simulink model "MINI_BANSHEE"  (Simulink 8.1)
settings: Solver=ode1  StartTime=0.0  StopTime=inf  FixedStep=Ts  MaxStep=1e-3  RelTol=1e-3
model workspace (MAT data in the model file):
  op_snapshot1 : opcond.OperatingPoint (value not decoded)
PostLoadFcn:
  | BANSHEE_init;
InitFcn:
  | BANSHEE_init;
undefined symbols (not defined in the file): cable_spec, F1, F2, F3, fdesignblkfcn, gcbh, Left, SM_UtilityService, Ts, type, utility_service_lib, V
libraries: rtio_generic_modbus x21, relay_modbus_lib x20, cables_lib x19, breaker_lib x18, rtio_opalrt_common x15, rtlab x14, simulink x10, artemis x7, transformer_lib x7, simulink_extras x6, PQFV_lib x5, rtio_opalrt_op5142ex1 x4
(part 1 of 3)
settings Model: ARTEMISmethode_block_infos=$$__separator__$$MINI_BANSHEE/ARTEMIS Guide$$__separator__$$  Creator=RE25624  LastModifiedBy=re25624  BufferReuse=off
settings SolverCC: ZeroCrossAlgorithm=Adaptive
settings DataIOCC: ExternalInput=getinputstruct(op_snapshot1)  InitialState=getstatestruct(op_snapshot1)  LimitDataPoints=off  MaxDataPoints=90060  SignalLoggingSaveFormat=Dataset  SaveOutput=off  SignalLogging=off  DSMLogging=off  SaveTime=off  OutputSaveName=result
settings OptimizationCC: BlockReduction=off  OptimizeBlockIOStorage=off  BufferReuse=off  ExpressionFolding=off  LocalBlockOutputs=off
settings DebuggingCC: MaxConsecutiveZCsMsg=warning  IgnoredZcDiagnostic=none  SolverPrmCheckMsg=none  MultiTaskRateTransMsg=warning  FcnCallInpInsideContextMsg=EnableAllAsWarning  FrameProcessingCompatibilityMsg=error  ModelReferenceExtraNoncontSigs=warning  StrictBusMsg=None
settings ModelReferenceCC: UpdateModelReferenceTargets=IfOutOfDate
settings SFSimCC: SFSimEcho=off
settings GRTTargetCC: CodeReplacementLibrary=C89/C90 (ANSI)

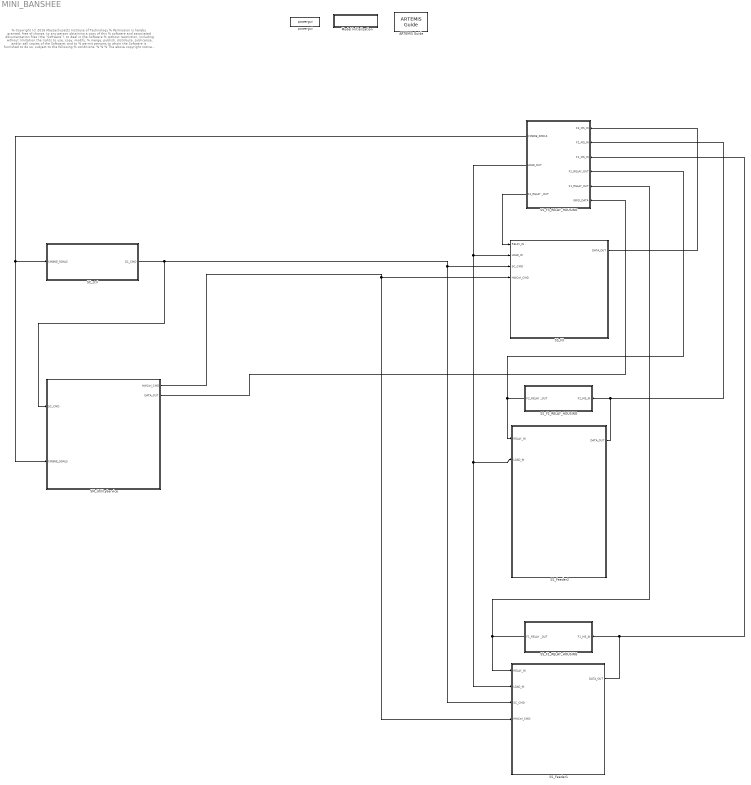
== system MINI_BANSHEE ==
  note: % Copyright (c) 2016 Massachusetts Institute of Technology
      | % Permission is hereby granted, free of charge, to any person obtaining a copy of this
      | % software and associated documentation files (the "Software"), to deal in the Software
      | % without restriction, including without limitation the rights to use, copy, modify,
      | % merge, publish, distribute, sublicense, and/or sell copies of the Software, and to
      | % permit persons to whom the Software is furnished to do so, subject to the following
      | % conditions:
      | %
      | %
      | % The above copyright notice and this permission notice shall be included in
      | % all copies or substantial portions of the Software.
      | %
      | % THE SOFTWARE IS PROVIDED "AS IS", WITHOUT WARRANTY OF ANY KIND, EXPRESS OR IMPLIED,
      | % INCLUDING BUT NOT LIMITED TO THE WARRANTIES OF MERCHANTABILITY, FITNESS FOR A
      | % PARTICULAR PURPOSE AND NONINFRINGEMENT. IN NO EVENT SHALL THE AUTHORS OR COPYRIGHT
      | % HOLDERS BE LIABLE FOR ANY CLAIM, DAMAGES OR OTHER LIABILITY, WHETHER IN AN ACTION
      | % OF CONTRACT, TORT OR OTHERWISE, ARISING FROM, OUT OF OR IN CONNECTION WITH THE
      | % SOFTWARE OR THE USE OR OTHER DEALINGS IN THE SOFTWARE.
      | %
      | %
      | %%
  ARTEMIS Guide : artemis/ARTEMIS/ARTEMIS Guide  Tag=FTSSmethode_opal_4hx0r99  Description=5.0_z1  lock=on  Ts=Ts  opt=art5  dyna=off  nb_perm=4  RT_fullcomp=off  ssn=on  ssn_itvc=off  ssn_ivic=off  ssn_ext=off  ssn_solver=Art5 with Backward Euler nodal interface  ssn_impulse=off  ssn_quasimpulse=off  ssn_impulse_loop=5  paraExtinctionThy=off  Thy_Impulse=on  dtc=Off  dtc_opt=normal  ao=on  simtype=off  ct_mac=off  lin_mov=off  lsp=[0.001 2]  spike_skip=Disabled  dtc_extra=1  dtc_sws=normal  dtc_pied=0.5  SPSRulesBlock=SPSRules  tre=on  ctmm=off  LF=off  dpl_type=ARTEMiS DPL  rlc_type=off  custom_type=off  para=on  ssn_ImpulseLoopBlockedStateUpdate=5  ssn_mov_iter_number=5  ssn_switch_iter_number=5
  Model Initialization : Subsystem  AncestorBlock=artemis/Tools /Misc/Model Initialization  mask(Model Functions){InitFcnX=BANSHEE_init;, prel=off, posl=on, inif=on, strf=off}
      mask prompts: InitFcnX "Initialisation"; prel "Preload Function"; posl "PostLoad Function"; inif "InitFcn"; strf "StartFcn"
      mask init:
      | currentBlock = gcb;
      | root = bdroot(currentBlock);
      | 
      | if ~strcmp(get_param(root,'BlockDiagramType'),'library')
      |     if prel==1
      |         set_param(root, 'PreLoadFcn', InitFcnX);
      |     else
      |         set_param(root, 'PreLoadFcn', '');
      |     end
      |     if inif==1
      |         set_param(root, 'InitFcn', InitFcnX);
      |     else
      |         set_param(root, 'InitFcn', '');
      |     end
      |     if strf==1
      |         set_param(root, 'StartFcn', InitFcnX);
      |     else
      |         set_param(root, 'StartFcn', '');
      |     end
      |     if posl==1
      |         set_param(root, 'PostLoadFcn', InitFcnX);
      |     else
      |         set_param(root, 'PostLoadFcn', '');
      |     end
      | end
      | 
      | pos = get_param(currentBlock, 'Position');
      | width = pos(3) - pos(1); height = pos(4) - pos(2);
      | txt = [ upper(root) '\n' '- InitFcn. . . . . '  get_param(root, 'InitFcn') ];
      settings: CopyFcn=set_param(gcb,'LinkStatus','inactive')
      mask Display: text(5, height*0.5, txt, 'horizontalAlignment', 'left', 'verticalAlignment', 'middle') ;
  SC_ctrl : Subsystem
  SM_UtilityService : Subsystem  AncestorBlock=utility_service_lib/SM_UtilityService
  SS_F1_RELAY_HOUSING : Subsystem
  SS_F2_RELAY_HOUSING : Subsystem
  SS_F3 : Subsystem
  SS_F3_RELAY_HOUSING : Subsystem
  SS_Feeder1 : Subsystem
  SS_Feeder2 : Subsystem
  powergui : powerlib/powergui  Priority=2  SimulationMode=Discrete  SolverType=Tustin  SampleTime=Ts  frequency=60  SPID=off  DisableSnubberDevices=off  DisableRonSwitches=off  DisableVfSwitches=off  SwTol=0  Interpol=off  DisplayEquations=off  frequencyindice=0  Pbase=100e6  ErrMax=1e-4  Iterations=50  UnitsV=kV  UnitsW=MW  FunctionMessages=off  echomessages=off  HookPort=off  EnableUseOfTLC=off  x0status=blocks  RestoreLinks=warning  ResistiveCurrentMeasurement=off  Frange=logspace(0,3,50)  Ylog=off  Xlog=off  ShowGrid=off  save=off  variable=ZData  structure=0  ZoomFFT=on  StartTime=0.0  cycles=2  DisplayStyle=off  fundamental=60  FreqAxis=off  MaxFrequency=1000  frequencyindicesteady=1  RmsSteady=1  display=off  Ts=0  methode=off
  wires:
  SS_F3/1(DATA_OUT) -> SS_F3_RELAY_HOUSING/1(F3_MS_IN)
  SS_F3_RELAY_HOUSING/3(F3_RELAY _OUT) -> SS_F3/1(RELAY_IN)
  SS_F1_RELAY_HOUSING/1(F1_RELAY _OUT) -> SS_Feeder1/1(RELAY_IN), SS_F3_RELAY_HOUSING/5(F1_RELAY_OUT)
  SS_F2_RELAY_HOUSING/1(F2_RELAY _OUT) -> SS_F3_RELAY_HOUSING/4(F2_RELAY_OUT), SS_Feeder2/1(RELAY_IN)
  SS_Feeder1/1(DATA_OUT) -> SS_F3_RELAY_HOUSING/3(F1_MS_IN), SS_F1_RELAY_HOUSING/1(F1_MS_IN)
  SS_Feeder2/1(DATA_OUT) -> SS_F3_RELAY_HOUSING/2(F2_MS_IN), SS_F2_RELAY_HOUSING/1(F2_MS_IN)
  SM_UtilityService/2(DATA_OUT) -> SS_F3_RELAY_HOUSING/6(GRID_DATA)
  SC_ctrl/1(SC_CMD) -> SM_UtilityService/1(SC_CMD), SS_Feeder1/3(SC_CMD), SS_F3/3(SC_CMD)
  SS_F3_RELAY_HOUSING/2(LOAD_OUT) -> SS_F3/2(LOAD_IN), SS_Feeder1/2(LOAD_IN), SS_Feeder2/2(LOAD_IN)
  SM_UtilityService/1(HWCtrl_CMD) -> SS_Feeder1/4(HWCtrl_CMD), SS_F3/4(HWCtrl_CMD)
  SS_F3_RELAY_HOUSING/1(CMBNE_SGNLS) -> SM_UtilityService/2(CMBNE_SGNLS), SC_ctrl/1(CMBNE_SGNLS)

== system MINI_BANSHEE/Model Initialization ==

== system MINI_BANSHEE/SC_ctrl ==
  note: % Copyright (c) 2016 Massachusetts Institute of Technology
      | % Permission is hereby granted, free of charge, to any person obtaining a copy of this
      | % software and associated documentation files (the "Software"), to deal in the Software
      | % without restriction, including without limitation the rights to use, copy, modify,
      | % merge, publish, distribute, sublicense, and/or sell copies of the Software, and to
      | % permit persons to whom the Software is furnished to do so, subject to the following
      | % conditions:
      | %
      | %
      | % The above copyright notice and this permission notice shall be included in
      | % all copies or substantial portions of the Software.
      | %
      | % THE SOFTWARE IS PROVIDED "AS IS", WITHOUT WARRANTY OF ANY KIND, EXPRESS OR IMPLIED,
      | % INCLUDING BUT NOT LIMITED TO THE WARRANTIES OF MERCHANTABILITY, FITNESS FOR A
      | % PARTICULAR PURPOSE AND NONINFRINGEMENT. IN NO EVENT SHALL THE AUTHORS OR COPYRIGHT
      | % HOLDERS BE LIABLE FOR ANY CLAIM, DAMAGES OR OTHER LIABILITY, WHETHER IN AN ACTION
      | % OF CONTRACT, TORT OR OTHERWISE, ARISING FROM, OUT OF OR IN CONNECTION WITH THE
      | % SOFTWARE OR THE USE OR OTHER DEALINGS IN THE SOFTWARE.
      | %
      | %
      | %%
  note: The 'Overruns' value should remain at 0.
      | The 'Ttotal' value should be equal to the
      | model Fixed-Step size.
  CMBNE_SGNLS : Inport
  Bus Creator : BusCreator  Inputs=2
  Bus Creator1 : BusCreator  Inputs=3
  Bus Selector : BusSelector  OutputSignals=F1_RELAY_OUT,F2_RELAY_OUT,F3_RELAY_OUT
  F1 1: connect motor 0: disconnect motor1 : Constant  Value=0
  F3 1: connect motor 0: disconnect motor : Constant  Value=0
  OpComm : rtlab/OpComm  nbport=1  groupe_acq=1  subsys_rate=0  st=0  Synchronization=on  Interpolation=on  Threshold=1.0  Missed_Data=off  Sim_Time=off  Samples=off  dynSigOut=off  from_console=0  warning_done=off  writeOpCommFile=off  Offset=off
  Overall : Subsystem
  Status : Subsystem
  Woodward : Subsystem
  opElectricFaultSelector : artemis/Tools /POW faults/opElectricFaultSelector  phase_a=on  phase_b=on  phase_c=on  gnd_fault=on  Tacq=1  Tst=[0.1 0 10]  enable_POW=off  angle_POW=[15 0 10]  Tdr="[0.5 0  10]"  fault_location_menu=No fault  T_init=2
  SC_CMD : Outport
  wires:
  CMBNE_SGNLS/1 -> OpComm/1
  Bus Selector/1 -> Overall/1(F1), Status/1(F1)  "<F1_RELAY_OUT>"
  Bus Selector/2 -> Overall/2(F2), Status/2(F2)  "<F2_RELAY_OUT>"
  Bus Selector/3 -> Status/3(F3), Overall/3(F3)  "<F3_RELAY_OUT>"
  opElectricFaultSelector/1 -> [fault_cmd]
  Bus Creator1/1 -> SC_CMD/1
  [IO_ctrl] -> Bus Creator1/3  "IO ctrl"
  Woodward/1(IOctrl) -> [IO_ctrl]
  [fault_cmd] -> Bus Creator1/1  "fault_cmd"
  OpComm/1 -> Bus Selector/1
  Bus Creator/1 -> Bus Creator1/2  "motor_ONOFF"
  F3 1: connect motor 0: disconnect motor/1 -> Bus Creator/1  "F3_motor_ONOFF"
  F1 1: connect motor 0: disconnect motor1/1 -> Bus Creator/2  "F1_motor_ONOFF"

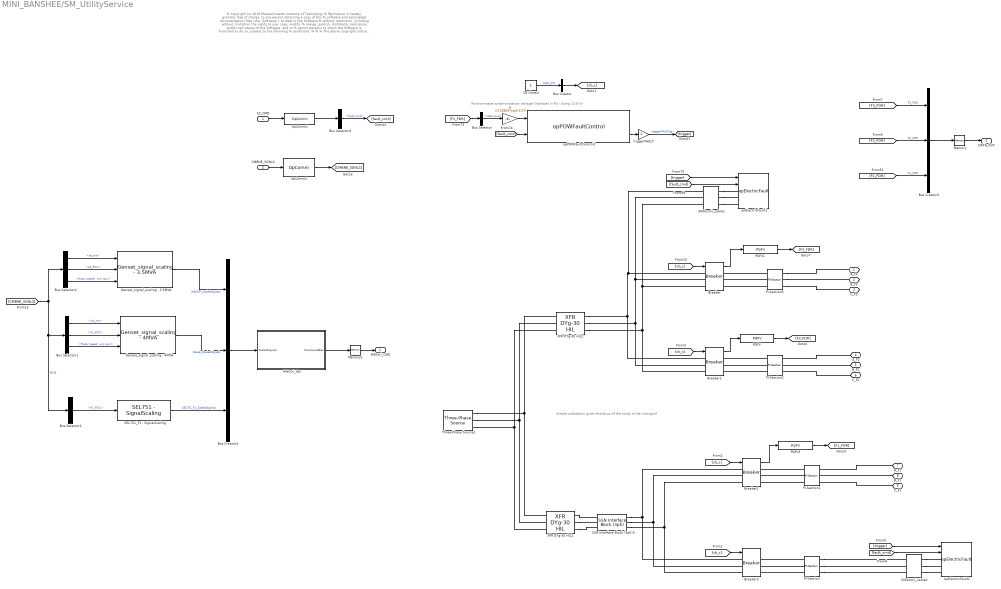
== system MINI_BANSHEE/SM_UtilityService ==
  note: Simple substation given the focus of the study is the microgrid
  note: % Copyright (c) 2016 Massachusetts Institute of Technology
      | % Permission is hereby granted, free of charge, to any person obtaining a copy of this
      | % software and associated documentation files (the "Software"), to deal in the Software
      | % without restriction, including without limitation the rights to use, copy, modify,
      | % merge, publish, distribute, sublicense, and/or sell copies of the Software, and to
      | % permit persons to whom the Software is furnished to do so, subject to the following
      | % conditions:
      | %
      | %
      | % The above copyright notice and this permission notice shall be included in
      | % all copies or substantial portions of the Software.
      | %
      | % THE SOFTWARE IS PROVIDED "AS IS", WITHOUT WARRANTY OF ANY KIND, EXPRESS OR IMPLIED,
      | % INCLUDING BUT NOT LIMITED TO THE WARRANTIES OF MERCHANTABILITY, FITNESS FOR A
      | % PARTICULAR PURPOSE AND NONINFRINGEMENT. IN NO EVENT SHALL THE AUTHORS OR COPYRIGHT
      | % HOLDERS BE LIABLE FOR ANY CLAIM, DAMAGES OR OTHER LIABILITY, WHETHER IN AN ACTION
      | % OF CONTRACT, TORT OR OTHERWISE, ARISING FROM, OUT OF OR IN CONNECTION WITH THE
      | % SOFTWARE OR THE USE OR OTHER DEALINGS IN THE SOFTWARE.
      | %
      | %
      | %%
  note: Point-on-wave synchronisation voltage (3-phase) in PU - Using 13.8 kV
  SC_CMD : Inport
  CMBNE_SGNLS : Inport  Port=2
  500kcmil_cable1 : cables_lib/500kcmil_cable  length=1  par_sets=1
  500kcmil_cable2 : cables_lib/500kcmil_cable  length=1  par_sets=1
  Breaker{,1..3} (4 alike) : breaker_lib/Breaker  Ts=Ts  mech_delay=cb_mech_delay
  Bus Creator : BusCreator  Inputs=1
  Bus Creator2 : BusCreator  Inputs=3
  Bus Creator4 : BusCreator  Inputs=3
  Bus Selector : BusSelector  OutputSignals=cb_ms.Vabc_bus
  Bus Selector1 : BusSelector  OutputSignals="F1_MS_IN.DIESEL_DATA.DIESEL_GCB.cb_ms,F1_MS_IN.CB_DATA.F1_PCC,F1_MS_IN.DIESEL_DATA.Gen2_meas.w.w.Rotor speed  wm (pu)"
  Bus Selector2 : BusSelector  OutputSignals=F1_MS_IN.CB_DATA.F1_PCC
  Bus Selector3 : BusSelector  OutputSignals=fault_cmd
  Bus Selector4 : BusSelector  OutputSignals="F3_MS_IN.NG_CHP_DATA.NG_CHP_GCB.cb_ms,F3_MS_IN.CB_DATA.F3_PCC,F3_MS_IN.NG_CHP_DATA.Gen1_meas.w.w.Rotor speed  wm (pu)"
  CB closed : Constant
  Genset_signal_scaling - 3.5MVA : EasyGen3500_GensetSignalScaling_lib/Genset_signal_scaling - 3.5MVA  Vpk_mcb=11268  watt_mcb=3150000  Vpk_gcb=11268  watt_gcb=3150000  rated_rpm=1800  wm_noise_bias=0.02
  Genset_signal_scaling - 4MVA : EasyGen3500_GensetSignalScaling_lib/Genset_signal_scaling - 4MVA  Vpk_mcb=11268  watt_mcb=3600000  Vpk_gcb=11268  watt_gcb=3600000  rated_rpm=1800  wm_noise_bias=0.02
  HWCtrl_IOs : Subsystem
  Memory : Memory
  Memory1 : Memory
  OpComm1 : rtlab/OpComm  nbport=1  groupe_acq=1  subsys_rate=0  st=0  Synchronization=on  Interpolation=on  Threshold=1.0  Missed_Data=off  Sim_Time=off  Samples=off  dynSigOut=off  from_console=1  warning_done=off  writeOpCommFile=off  Offset=off
  OpComm2 : rtlab/OpComm  nbport=1  groupe_acq=1  subsys_rate=0  st=0  Synchronization=on  Interpolation=on  Threshold=1.0  Missed_Data=off  Sim_Time=off  Samples=off  dynSigOut=off  from_console=0  warning_done=off  writeOpCommFile=off  Offset=off
  PI-Section : cables_lib/PI-Section  cable_spec=[cable_spec(13, :)]  line_length=3000  parallel_sets=1
  PI-Section1 : cables_lib/PI-Section  cable_spec=[cable_spec(13, :)]  line_length=500  parallel_sets=1
  PI-Section2 : cables_lib/PI-Section  cable_spec=[cable_spec(13, :)]  line_length=500  parallel_sets=1
  PI-Section3 : cables_lib/PI-Section  cable_spec=[cable_spec(13, :)]  line_length=500  parallel_sets=1
  PQFV : PQFV_lib/PQFV  VRMSLL=13800
  PQFV1 : PQFV_lib/PQFV  VRMSLL=13800
  PQFV3 : PQFV_lib/PQFV  VRMSLL=13800
  SEL751_F1 - SignalScaling : SEL751_SignalScaling_lib/SEL751 - SignalScaling  ct_ratio=1/1250  pt_ratio=1/1800
  SSN Interface Block (3ph)3 : ssn_lib/SSN Interface Block (3ph)  nb_phase=3  nb_port=2  p1_type=V-type(Left)  p2_type=V-type (Right)  p3_type=V-type(Left)  p4_type=V-type(Left)  p5_type=V-type(Left)  p6_type=V-type(Left)  p7_type=V-type(Left)  p8_type=V-type(Left)  p9_type=V-type(Left)  p10_type=V-type(Left)  p11_type=V-type(Left)  p12_type=V-type(Left)  p13_type=V-type(Left)  p14_type=V-type(Left)  p15_type=V-type(Left)  p16_type=V-type(Left)  I_port_shunt_resistance=1e9
  Three-Phase Source1 : powerlib/Electrical Sources/Three-Phase Source  Voltage=115000  PhaseAngle=0  Frequency=60  InternalConnection=Yg  SpecifyImpedance=on  Resistance=0.8929  Inductance=16.58e-3  ShortCircuitLevel=100e6  BaseVoltage=115000  XRratio=30  BusType=swing  Pref=0  Qref=0  Qmin=-inf  Qmax=inf
  XFR DYg-30 HIL1 : transformer_lib/XFR DYg-30 HIL  Rating=50000  Vp=115000  Vs=13800  Z=15  XR=30
  XFR DYg-30 HIL2 : transformer_lib/XFR DYg-30 HIL  Rating=50000  Vp=115000  Vs=13800  Z=15  XR=30
  a : Gain  Gain=1/(13800*sqrt(2/3))
  opElectricFault1 : artemis/Tools /POW faults/opElectricFault  FaultLocation=location 7  FaultResistance=0.0001  GroundResistance=0.0001  InitialStates=[0 0 0]  SnubberResistance=1e6  SnubberCapacitance=inf
  opElectricFault2 : artemis/Tools /POW faults/opElectricFault  FaultLocation=location 8  FaultResistance=0.0001  GroundResistance=0.0001  InitialStates=[0 0 0]  SnubberResistance=1e6  SnubberCapacitance=inf
  opPOWFaultControl1 : artemis/Tools /POW faults/opPOWFaultControl  Ts=Ts  usePLL=off  Fgrid=60  PLL_k=[180 3200 1]  vol_sel=1: rising zero-corssing  SyncPhase_menu=A  T_acq=0.8
  triggerFAULT : Gain
  A_F3 : PMIOPort  Port=1  Side=Right
  B_F3 : PMIOPort  Port=2  Side=Right
  C_F3 : PMIOPort  Port=3  Side=Right
  A_F2 : PMIOPort  Port=4  Side=Right
  B_F2 : PMIOPort  Port=5  Side=Right
  C_F2 : PMIOPort  Port=6  Side=Right
  A_F1 : PMIOPort  Port=7  Side=Right
  B_F1 : PMIOPort  Port=8  Side=Right
  C_F1 : PMIOPort  Port=9  Side=Right
  HWCtrl_CMD : Outport
  DATA_OUT : Outport  Port=2
  wires:
  [cb_c] -> Breaker2/1
  [cb_c] -> Breaker/1
  [cb_c] -> Breaker1/1
  [cb_c] -> Breaker3/1
  Bus Creator/1 -> [cb_c]
  CB closed/1 -> Bus Creator/1  "Logic_trip"
  [fault_cmd] -> opElectricFault1/2
  [trigger] -> opElectricFault1/1
  [fault_cmd] -> opPOWFaultControl1/2
  opPOWFaultControl1/2 -> triggerFAULT/1
  triggerFAULT/1 -> [trigger]  "triggerFAULTsig"
  [F1_FDR] -> Bus Selector/1
  Bus Selector/1 -> a/1  "<Vabc_bus>"
  a/1 -> opPOWFaultControl1/1
  [fault_cmd] -> opElectricFault2/2
  [trigger] -> opElectricFault2/1
  SC_CMD/1 -> OpComm1/1
  OpComm1/1 -> Bus Selector3/1
  Bus Selector3/1 -> [fault_cmd]  "<fault_cmd>"
  Memory1/1 -> HWCtrl_CMD/1
  Genset_signal_scaling - 3.5MVA/1 -> Bus Creator4/1  "NGCHP_ScaledSignals"
  Genset_signal_scaling - 4MVA/1 -> Bus Creator4/2  "Diesel_ScaledSignals"
  [CMBNE_SGNLS] -> Bus Selector4/1, Bus Selector2/1, Bus Selector1/1  "MCB"
  Bus Selector4/3 -> Genset_signal_scaling - 3.5MVA/3  "<Rotor speed  wm (pu)>"
  Bus Selector4/2 -> Genset_signal_scaling - 3.5MVA/2  "<F3_PCC>"
  Bus Selector4/1 -> Genset_signal_scaling - 3.5MVA/1  "<cb_ms>"
  Bus Creator4/1 -> HWCtrl_IOs/1(ScaledSignals)
  HWCtrl_IOs/1(WoodwardBias) -> Memory1/1
  Bus Selector1/3 -> Genset_signal_scaling - 4MVA/3  "<Rotor speed  wm (pu)>"
  Bus Selector1/2 -> Genset_signal_scaling - 4MVA/2  "<F1_PCC>"
  Bus Selector1/1 -> Genset_signal_scaling - 4MVA/1  "<cb_ms>"
  CMBNE_SGNLS/1 -> OpComm2/1
  OpComm2/1 -> [CMBNE_SGNLS]
  Breaker/1 -> PQFV1/1
  Breaker1/1 -> PQFV/1
  Breaker2/1 -> PQFV3/1
  PQFV3/1 -> [F1_FDR]
  PQFV1/1 -> [F3_FDR]
  PQFV/1 -> [F2_FDR]
  Memory/1 -> DATA_OUT/1
  Bus Creator2/1 -> Memory/1
  [F3_FDR] -> Bus Creator2/1  "F3_FDR"
  [F2_FDR] -> Bus Creator2/2  "F2_FDR"
  [F1_FDR] -> Bus Creator2/3  "F1_FDR"
  SEL751_F1 - SignalScaling/1 -> Bus Creator4/3  "SEL751_F1_ScaledSignals"
  Bus Selector2/1 -> SEL751_F1 - SignalScaling/1  "<F1_PCC>"
  connections:
  PI-Section2/LConn1 -- Breaker1/RConn1
  PI-Section2/LConn3 -- Breaker1/RConn3
  PI-Section1/LConn1 -- Breaker2/RConn1
  PI-Section1/LConn2 -- Breaker2/RConn2
  PI-Section3/LConn1 -- Breaker/RConn1
  PI-Section1/LConn3 -- Breaker2/RConn3
  Breaker3/LConn2 -- SSN Interface Block (3ph)3/RConn2 -- Breaker2/LConn2
  PI-Section3/LConn2 -- Breaker/RConn2
  Breaker3/LConn3 -- SSN Interface Block (3ph)3/RConn3 -- Breaker2/LConn3
  PI-Section/LConn3 -- Breaker3/RConn3
  PI-Section2/LConn2 -- Breaker1/RConn2
  PI-Section/LConn1 -- Breaker3/RConn1
  Breaker3/LConn1 -- SSN Interface Block (3ph)3/RConn1 -- Breaker2/LConn1
  PI-Section3/LConn3 -- Breaker/RConn3
  Breaker1/LConn2 -- 500kcmil_cable1/LConn2 -- Breaker/LConn2 -- XFR DYg-30 HIL2/RConn2
  XFR DYg-30 HIL2/RConn1 -- Breaker1/LConn1 -- 500kcmil_cable1/LConn1 -- Breaker/LConn1
  Breaker1/LConn3 -- 500kcmil_cable1/LConn3 -- Breaker/LConn3 -- XFR DYg-30 HIL2/RConn3
  PI-Section/LConn2 -- Breaker3/RConn2
  A_F2/RConn1 -- PI-Section2/RConn1
  B_F1/RConn1 -- PI-Section1/RConn2
  PI-Section3/RConn3 -- C_F3/RConn1
  Three-Phase Source1/RConn3 -- XFR DYg-30 HIL2/LConn3 -- XFR DYg-30 HIL1/LConn3
  Three-Phase Source1/RConn2 -- XFR DYg-30 HIL2/LConn2 -- XFR DYg-30 HIL1/LConn2
  Three-Phase Source1/RConn1 -- XFR DYg-30 HIL2/LConn1 -- XFR DYg-30 HIL1/LConn1
  C_F2/RConn1 -- PI-Section2/RConn3
  PI-Section3/RConn1 -- A_F3/RConn1
  B_F2/RConn1 -- PI-Section2/RConn2
  A_F1/RConn1 -- PI-Section1/RConn1
  C_F1/RConn1 -- PI-Section1/RConn3
  PI-Section3/RConn2 -- B_F3/RConn1
  500kcmil_cable1/RConn3 -- opElectricFault1/LConn3
  500kcmil_cable1/RConn2 -- opElectricFault1/LConn2
  500kcmil_cable1/RConn1 -- opElectricFault1/LConn1
  500kcmil_cable2/RConn3 -- opElectricFault2/LConn3
  500kcmil_cable2/RConn2 -- opElectricFault2/LConn2
  500kcmil_cable2/RConn1 -- opElectricFault2/LConn1
  PI-Section/RConn3 -- 500kcmil_cable2/LConn3
  PI-Section/RConn2 -- 500kcmil_cable2/LConn2
  PI-Section/RConn1 -- 500kcmil_cable2/LConn1
  XFR DYg-30 HIL1/RConn3 -- SSN Interface Block (3ph)3/LConn3
  XFR DYg-30 HIL1/RConn2 -- SSN Interface Block (3ph)3/LConn2
  XFR DYg-30 HIL1/RConn1 -- SSN Interface Block (3ph)3/LConn1

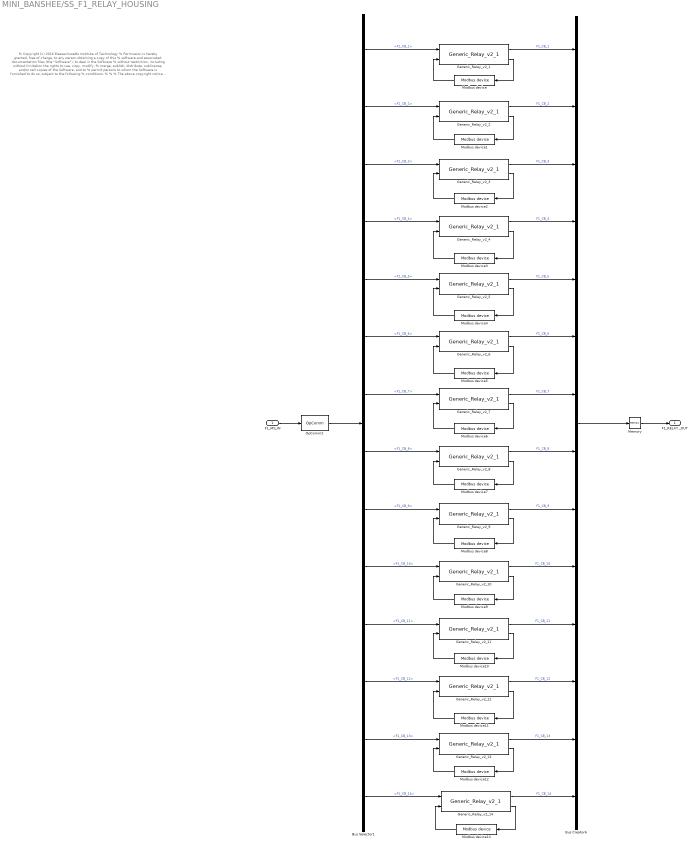
== system MINI_BANSHEE/SS_F1_RELAY_HOUSING ==
  note: % Copyright (c) 2016 Massachusetts Institute of Technology
      | % Permission is hereby granted, free of charge, to any person obtaining a copy of this
      | % software and associated documentation files (the "Software"), to deal in the Software
      | % without restriction, including without limitation the rights to use, copy, modify,
      | % merge, publish, distribute, sublicense, and/or sell copies of the Software, and to
      | % permit persons to whom the Software is furnished to do so, subject to the following
      | % conditions:
      | %
      | %
      | % The above copyright notice and this permission notice shall be included in
      | % all copies or substantial portions of the Software.
      | %
      | % THE SOFTWARE IS PROVIDED "AS IS", WITHOUT WARRANTY OF ANY KIND, EXPRESS OR IMPLIED,
      | % INCLUDING BUT NOT LIMITED TO THE WARRANTIES OF MERCHANTABILITY, FITNESS FOR A
      | % PARTICULAR PURPOSE AND NONINFRINGEMENT. IN NO EVENT SHALL THE AUTHORS OR COPYRIGHT
      | % HOLDERS BE LIABLE FOR ANY CLAIM, DAMAGES OR OTHER LIABILITY, WHETHER IN AN ACTION
      | % OF CONTRACT, TORT OR OTHERWISE, ARISING FROM, OUT OF OR IN CONNECTION WITH THE
      | % SOFTWARE OR THE USE OR OTHER DEALINGS IN THE SOFTWARE.
      | %
      | %
      | %%
  F1_MS_IN : Inport
  Bus Creator6 : BusCreator  Inputs=14
  Bus Selector1 : BusSelector  OutputSignals=CB_DATA.F1_CB_1,CB_DATA.F1_CB_2,CB_DATA.F1_CB_3,CB_DATA.F1_CB_4,CB_DATA.F1_CB_5,CB_DATA.F1_CB_6,CB_DATA.F1_CB_7,CB_DATA.F1_CB_8,CB_DATA.F1_CB_9,CB_DATA.F1_CB_10,CB_DATA.F1_CB_11,CB_DATA.F1_CB_12,CB_DATA.F1_CB_13,CB_DATA.F1_CB_14
  Generic_Relay_v2_1 : relay_modbus_lib/Generic_Relay_v2_1  Ts=Ts  relay_settings=[F1(1,:)]
  Generic_Relay_v2_10 : relay_modbus_lib/Generic_Relay_v2_1  Ts=Ts  relay_settings=[F1(10,:)]
  Generic_Relay_v2_11 : relay_modbus_lib/Generic_Relay_v2_1  Ts=Ts  relay_settings=[F1(11,:)]
  Generic_Relay_v2_12 : relay_modbus_lib/Generic_Relay_v2_1  Ts=Ts  relay_settings=[F1(12,:)]
  Generic_Relay_v2_13 : relay_modbus_lib/Generic_Relay_v2_1  Ts=Ts  relay_settings=[F1(13,:)]
  Generic_Relay_v2_14 : relay_modbus_lib/Generic_Relay_v2_1  Ts=Ts  relay_settings=[F1(14,:)]
  Generic_Relay_v2_2 : relay_modbus_lib/Generic_Relay_v2_1  Ts=Ts  relay_settings=[F1(2,:)]
  Generic_Relay_v2_3 : relay_modbus_lib/Generic_Relay_v2_1  Ts=Ts  relay_settings=[F1(3,:)]
  Generic_Relay_v2_4 : relay_modbus_lib/Generic_Relay_v2_1  Ts=Ts  relay_settings=[F1(4,:)]
  Generic_Relay_v2_5 : relay_modbus_lib/Generic_Relay_v2_1  Ts=Ts  relay_settings=[F1(5,:)]
  Generic_Relay_v2_6 : relay_modbus_lib/Generic_Relay_v2_1  Ts=Ts  relay_settings=[F1(6,:)]
  Generic_Relay_v2_7 : relay_modbus_lib/Generic_Relay_v2_1  Ts=Ts  relay_settings=[F1(7,:)]
  Generic_Relay_v2_8 : relay_modbus_lib/Generic_Relay_v2_1  Ts=Ts  relay_settings=[F1(8,:)]
  Generic_Relay_v2_9 : relay_modbus_lib/Generic_Relay_v2_1  Ts=Ts  relay_settings=[F1(9,:)]
  Memory : Memory
  Modbus device : rtio_generic_modbus/Modbus device  conf_name=F1_relay_cfg1.opal  conf_name_mask=F1_relay_cfg1.xls  sample_time=Ts
  Modbus device1 : rtio_generic_modbus/Modbus device  conf_name=F1_relay_cfg2.opal  conf_name_mask=F1_relay_cfg2.xls  sample_time=Ts
  Modbus device10 : rtio_generic_modbus/Modbus device  conf_name=F1_relay_cfg11.opal  conf_name_mask=F1_relay_cfg11.xls  sample_time=Ts
  Modbus device11 : rtio_generic_modbus/Modbus device  conf_name=F1_relay_cfg12.opal  conf_name_mask=F1_relay_cfg12.xls  sample_time=Ts
  Modbus device12 : rtio_generic_modbus/Modbus device  conf_name=F1_relay_cfg13.opal  conf_name_mask=F1_relay_cfg13.xls  sample_time=Ts
  Modbus device13 : rtio_generic_modbus/Modbus device  conf_name=F1_relay_cfg14.opal  conf_name_mask=F1_relay_cfg14.xls  sample_time=Ts
  Modbus device2 : rtio_generic_modbus/Modbus device  conf_name=F1_relay_cfg3.opal  conf_name_mask=F1_relay_cfg3.xls  sample_time=Ts
  Modbus device3 : rtio_generic_modbus/Modbus device  conf_name=F1_relay_cfg4.opal  conf_name_mask=F1_relay_cfg4.xls  sample_time=Ts
  Modbus device4 : rtio_generic_modbus/Modbus device  conf_name=F1_relay_cfg5.opal  conf_name_mask=F1_relay_cfg5.xls  sample_time=Ts
  Modbus device5 : rtio_generic_modbus/Modbus device  conf_name=F1_relay_cfg6.opal  conf_name_mask=F1_relay_cfg6.xls  sample_time=Ts
  Modbus device6 : rtio_generic_modbus/Modbus device  conf_name=F1_relay_cfg7.opal  conf_name_mask=F1_relay_cfg7.xls  sample_time=Ts
  Modbus device7 : rtio_generic_modbus/Modbus device  conf_name=F1_relay_cfg8.opal  conf_name_mask=F1_relay_cfg8.xls  sample_time=Ts
  Modbus device8 : rtio_generic_modbus/Modbus device  conf_name=F1_relay_cfg9.opal  conf_name_mask=F1_relay_cfg9.xls  sample_time=Ts
  Modbus device9 : rtio_generic_modbus/Modbus device  conf_name=F1_relay_cfg10.opal  conf_name_mask=F1_relay_cfg10.xls  sample_time=Ts
  OpComm2 : rtlab/OpComm  nbport=1  groupe_acq=1  subsys_rate=0  st=0  Synchronization=on  Interpolation=on  Threshold=1.0  Missed_Data=off  Sim_Time=off  Samples=off  dynSigOut=off  from_console=0  warning_done=off  writeOpCommFile=off  Offset=off
  F1_RELAY _OUT : Outport
  wires:
  OpComm2/1 -> Bus Selector1/1
  Modbus device12/1 -> Generic_Relay_v2_13/2
  Generic_Relay_v2_13/2 -> Modbus device12/1
  Modbus device11/1 -> Generic_Relay_v2_12/2
  Generic_Relay_v2_12/2 -> Modbus device11/1
  Modbus device10/1 -> Generic_Relay_v2_11/2
  Generic_Relay_v2_11/2 -> Modbus device10/1
  Modbus device9/1 -> Generic_Relay_v2_10/2
  Generic_Relay_v2_10/2 -> Modbus device9/1
  Modbus device8/1 -> Generic_Relay_v2_9/2
  Generic_Relay_v2_9/2 -> Modbus device8/1
  Modbus device7/1 -> Generic_Relay_v2_8/2
  Generic_Relay_v2_8/2 -> Modbus device7/1
  Modbus device6/1 -> Generic_Relay_v2_7/2
  Generic_Relay_v2_7/2 -> Modbus device6/1
  Modbus device5/1 -> Generic_Relay_v2_6/2
  Generic_Relay_v2_6/2 -> Modbus device5/1
  Modbus device4/1 -> Generic_Relay_v2_5/2
  Generic_Relay_v2_5/2 -> Modbus device4/1
  Modbus device3/1 -> Generic_Relay_v2_4/2
  Generic_Relay_v2_4/2 -> Modbus device3/1
  Modbus device2/1 -> Generic_Relay_v2_3/2
  Generic_Relay_v2_3/2 -> Modbus device2/1
  Generic_Relay_v2_2/2 -> Modbus device1/1
  Modbus device1/1 -> Generic_Relay_v2_2/2
  Generic_Relay_v2_1/2 -> Modbus device/1
  Modbus device/1 -> Generic_Relay_v2_1/2
  F1_MS_IN/1 -> OpComm2/1
  Bus Selector1/1 -> Generic_Relay_v2_1/1  "<F1_CB_1>"
  Generic_Relay_v2_1/1 -> Bus Creator6/1  "F1_CB_1"
  Bus Creator6/1 -> Memory/1
  Bus Selector1/2 -> Generic_Relay_v2_2/1  "<F1_CB_2>"
  Generic_Relay_v2_2/1 -> Bus Creator6/2  "F1_CB_2"
  Bus Selector1/3 -> Generic_Relay_v2_3/1  "<F1_CB_3>"
  Bus Selector1/4 -> Generic_Relay_v2_4/1  "<F1_CB_4>"
  Bus Selector1/5 -> Generic_Relay_v2_5/1  "<F1_CB_5>"
  Bus Selector1/6 -> Generic_Relay_v2_6/1  "<F1_CB_6>"
  Bus Selector1/7 -> Generic_Relay_v2_7/1  "<F1_CB_7>"
  Bus Selector1/8 -> Generic_Relay_v2_8/1  "<F1_CB_8>"
  Bus Selector1/9 -> Generic_Relay_v2_9/1  "<F1_CB_9>"
  Bus Selector1/10 -> Generic_Relay_v2_10/1  "<F1_CB_10>"
  Bus Selector1/11 -> Generic_Relay_v2_11/1  "<F1_CB_11>"
  Bus Selector1/12 -> Generic_Relay_v2_12/1  "<F1_CB_12>"
  Bus Selector1/13 -> Generic_Relay_v2_13/1  "<F1_CB_13>"
  Generic_Relay_v2_13/1 -> Bus Creator6/13  "F1_CB_13"
  Generic_Relay_v2_12/1 -> Bus Creator6/12  "F1_CB_12"
  Generic_Relay_v2_11/1 -> Bus Creator6/11  "F1_CB_11"
  Generic_Relay_v2_10/1 -> Bus Creator6/10  "F1_CB_10"
  Generic_Relay_v2_9/1 -> Bus Creator6/9  "F1_CB_9"
  Generic_Relay_v2_8/1 -> Bus Creator6/8  "F1_CB_8"
  Generic_Relay_v2_7/1 -> Bus Creator6/7  "F1_CB_7"
  Generic_Relay_v2_6/1 -> Bus Creator6/6  "F1_CB_6"
  Generic_Relay_v2_5/1 -> Bus Creator6/5  "F1_CB_5"
  Generic_Relay_v2_4/1 -> Bus Creator6/4  "F1_CB_4"
  Generic_Relay_v2_3/1 -> Bus Creator6/3  "F1_CB_3"
  Modbus device13/1 -> Generic_Relay_v2_14/2
  Generic_Relay_v2_14/2 -> Modbus device13/1
  Generic_Relay_v2_14/1 -> Bus Creator6/14  "F1_CB_14"
  Bus Selector1/14 -> Generic_Relay_v2_14/1  "<F1_CB_14>"
  Memory/1 -> F1_RELAY _OUT/1

== system MINI_BANSHEE/SS_F2_RELAY_HOUSING ==
  note: % Copyright (c) 2016 Massachusetts Institute of Technology
      | % Permission is hereby granted, free of charge, to any person obtaining a copy of this
      | % software and associated documentation files (the "Software"), to deal in the Software
      | % without restriction, including without limitation the rights to use, copy, modify,
      | % merge, publish, distribute, sublicense, and/or sell copies of the Software, and to
      | % permit persons to whom the Software is furnished to do so, subject to the following
      | % conditions:
      | %
      | %
      | % The above copyright notice and this permission notice shall be included in
      | % all copies or substantial portions of the Software.
      | %
      | % THE SOFTWARE IS PROVIDED "AS IS", WITHOUT WARRANTY OF ANY KIND, EXPRESS OR IMPLIED,
      | % INCLUDING BUT NOT LIMITED TO THE WARRANTIES OF MERCHANTABILITY, FITNESS FOR A
      | % PARTICULAR PURPOSE AND NONINFRINGEMENT. IN NO EVENT SHALL THE AUTHORS OR COPYRIGHT
      | % HOLDERS BE LIABLE FOR ANY CLAIM, DAMAGES OR OTHER LIABILITY, WHETHER IN AN ACTION
      | % OF CONTRACT, TORT OR OTHERWISE, ARISING FROM, OUT OF OR IN CONNECTION WITH THE
      | % SOFTWARE OR THE USE OR OTHER DEALINGS IN THE SOFTWARE.
      | %
      | %
      | %%
  F2_MS_IN : Inport
  Bus Creator6 : BusCreator  Inputs=19
  Bus Selector2 : BusSelector  OutputSignals=CB_DATA.F2_CB_1,CB_DATA.F2_CB_2,CB_DATA.F2_CB_3,CB_DATA.F2_CB_4,CB_DATA.F2_CB_5,CB_DATA.F2_CB_6,CB_DATA.F2_CB_7,CB_DATA.F2_CB_8,CB_DATA.F2_CB_9,CB_DATA.F2_CB_10,CB_DATA.F2_CB_11,CB_DATA.F2_CB_12,CB_DATA.F2_CB_13,CB_DATA.F2_CB_14,CB_DATA.F2_CB_15,CB_DATA.F2_CB_16,CB_DATA.F2_CB_17,CB_DATA.F2_CB_18,CB_DATA.F2_CB_19
  Generic_Relay_v2_1 : relay_modbus_lib/Generic_Relay_v2_1  Ts=Ts  relay_settings=[F2(1,:)]
  Generic_Relay_v2_2 : relay_modbus_lib/Generic_Relay_v2_1  Ts=Ts  relay_settings=[F2(2,:)]
  Generic_Relay_v2_3 : relay_modbus_lib/Generic_Relay_v2_1  Ts=Ts  relay_settings=[F2(3,:)]
  Memory : Memory
  Modbus device : rtio_generic_modbus/Modbus device  conf_name=F2_relay_cfg1.opal  conf_name_mask=F2_relay_cfg1.xls  sample_time=Ts
  Modbus device1 : rtio_generic_modbus/Modbus device  conf_name=F2_relay_cfg2.opal  conf_name_mask=F2_relay_cfg2.xls  sample_time=Ts
  Modbus device2 : rtio_generic_modbus/Modbus device  conf_name=F2_relay_cfg3.opal  conf_name_mask=F2_relay_cfg3.xls  sample_time=Ts
  OpComm2 : rtlab/OpComm  nbport=1  groupe_acq=1  subsys_rate=0  st=0  Synchronization=on  Interpolation=on  Threshold=1.0  Missed_Data=off  Sim_Time=off  Samples=off  dynSigOut=off  from_console=0  warning_done=off  writeOpCommFile=off  Offset=off
  F2_RELAY _OUT : Outport
  wires:
  OpComm2/1 -> Bus Selector2/1
  Modbus device2/1 -> Generic_Relay_v2_3/2
  Generic_Relay_v2_3/2 -> Modbus device2/1
  Modbus device1/1 -> Generic_Relay_v2_2/2
  Generic_Relay_v2_2/2 -> Modbus device1/1
  Modbus device/1 -> Generic_Relay_v2_1/2
  Generic_Relay_v2_1/2 -> Modbus device/1
  Bus Creator6/1 -> Memory/1
  F2_MS_IN/1 -> OpComm2/1
  Bus Selector2/1 -> Generic_Relay_v2_1/1  "<F2_CB_1>"
  Generic_Relay_v2_1/1 -> Bus Creator6/1  "F2_CB_1"
  Bus Selector2/2 -> Generic_Relay_v2_2/1  "<F2_CB_2>"
  Bus Selector2/3 -> Generic_Relay_v2_3/1  "<F2_CB_3>"
  Generic_Relay_v2_2/1 -> Bus Creator6/2  "F2_CB_2"
  Generic_Relay_v2_3/1 -> Bus Creator6/3  "F2_CB_3"
  Memory/1 -> F2_RELAY _OUT/1

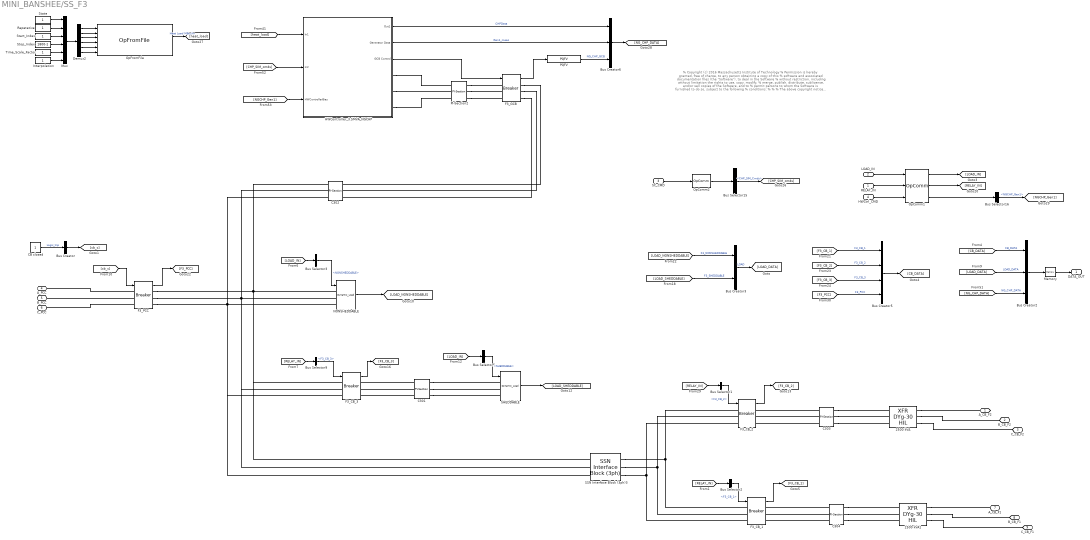
== system MINI_BANSHEE/SS_F3 ==
  note: % Copyright (c) 2016 Massachusetts Institute of Technology
      | % Permission is hereby granted, free of charge, to any person obtaining a copy of this
      | % software and associated documentation files (the "Software"), to deal in the Software
      | % without restriction, including without limitation the rights to use, copy, modify,
      | % merge, publish, distribute, sublicense, and/or sell copies of the Software, and to
      | % permit persons to whom the Software is furnished to do so, subject to the following
      | % conditions:
      | %
      | %
      | % The above copyright notice and this permission notice shall be included in
      | % all copies or substantial portions of the Software.
      | %
      | % THE SOFTWARE IS PROVIDED "AS IS", WITHOUT WARRANTY OF ANY KIND, EXPRESS OR IMPLIED,
      | % INCLUDING BUT NOT LIMITED TO THE WARRANTIES OF MERCHANTABILITY, FITNESS FOR A
      | % PARTICULAR PURPOSE AND NONINFRINGEMENT. IN NO EVENT SHALL THE AUTHORS OR COPYRIGHT
      | % HOLDERS BE LIABLE FOR ANY CLAIM, DAMAGES OR OTHER LIABILITY, WHETHER IN AN ACTION
      | % OF CONTRACT, TORT OR OTHERWISE, ARISING FROM, OUT OF OR IN CONNECTION WITH THE
      | % SOFTWARE OR THE USE OR OTHER DEALINGS IN THE SOFTWARE.
      | %
      | %
      | %%
  RELAY_IN : Inport
  LOAD_IN : Inport  Port=2
  SC_CMD : Inport  Port=3
  HWCtrl_CMD : Inport  Port=4
  2500 kVA : transformer_lib/XFR DYg-30 HIL  Rating=2500  Vp=13800  Vs=480  Z=5.75  XR=6.6
  2500 kVA1 : transformer_lib/XFR DYg-30 HIL  Rating=2500  Vp=13800  Vs=480  Z=5.75  XR=6.6
  Bus Creator : BusCreator  Inputs=1
  Bus Creator2 : BusCreator  Inputs=3
  Bus Creator3 : BusCreator  Inputs=2
  Bus Creator5 : BusCreator
  Bus Creator6 : BusCreator  Inputs=3
  Bus Selector1 : BusSelector  OutputSignals=F3_CB_2
  Bus Selector15 : BusSelector  OutputSignals=IO ctrl.16 DOUT GR3.CHP_SIM_Cmds
  Bus Selector16 : BusSelector  OutputSignals=NGCHP_Gen1
  Bus Selector2 : BusSelector  OutputSignals=F3_CB_1
  Bus Selector3 : BusSelector  OutputSignals=NONSHEDDABLE
  Bus Selector5 : BusSelector  OutputSignals=SHEDDABLE
  Bus Selector9 : BusSelector  OutputSignals=F3_CB_3
  C301 : cables_lib/PI-Section  cable_spec=[cable_spec(13, :)]  line_length=2500  parallel_sets=1
  C302 : cables_lib/PI-Section  cable_spec=[cable_spec(11, :)]  line_length=2000  parallel_sets=1
  C303 : cables_lib/PI-Section  cable_spec=[cable_spec(13, :)]  line_length=2000  parallel_sets=1
  C304 : cables_lib/PI-Section  cable_spec=[cable_spec(13, :)]  line_length=2000  parallel_sets=1
  CB closed : Constant
  Demux2 : Demux  Outputs=6
  F3_CB_1 : breaker_lib/Breaker  Ts=Ts  mech_delay=cb_mech_delay
  F3_CB_2 : breaker_lib/Breaker  Ts=Ts  mech_delay=cb_mech_delay
  F3_CB_3 : breaker_lib/Breaker  Ts=Ts  mech_delay=cb_mech_delay
  F3_GCB : breaker_lib/Breaker  Ts=Ts  mech_delay=cb_mech_delay
  F3_PCC : breaker_lib/Breaker  Ts=Ts  mech_delay=cb_mech_delay
  HWController_3.5MVA_NGCHP : Subsystem  AncestorBlock=HWController_NGCHP_Genset_3p5MVA_lib/HWController_3.5MVA_NGCHP
  "Interpolation " : Constant
  Memory : Memory
  Mux : Mux  Inputs=6
  NONSHEDDABLE : Load_lib/Dynamic_Load  V=13800  Ts=Ts
  OpComm1 : rtlab/OpComm  nbport=3  groupe_acq=1  subsys_rate=0  st=0  Synchronization=on  Interpolation=on  Threshold=1.0  Missed_Data=off  Sim_Time=off  Samples=off  dynSigOut=off  from_console=0  warning_done=off  writeOpCommFile=off  Offset=off
  OpComm2 : rtlab/OpComm  nbport=1  groupe_acq=1  subsys_rate=0  st=0  Synchronization=on  Interpolation=on  Threshold=1.0  Missed_Data=off  Sim_Time=off  Samples=off  dynSigOut=off  from_console=1  warning_done=off  writeOpCommFile=off  Offset=off
  OpFromFile : rtlab/DataLogging/OpFromFile  filename_mode=Static (same filename all the time)  reload_mode=Next time model is paused (Real-Time)  init_file_id=0  filename=HeatLoad.mat  rtpath='./'  nrtpath='.\'  sample_time=Ts
  PI-Section2 : cables_lib/PI-Section  cable_spec=[cable_spec(11, :)]  line_length=2000  parallel_sets=1
  PQFV : PQFV_lib/PQFV  VRMSLL=13800
  "Repetative " : Constant
  SHEDDABLE : Load_lib/Dynamic_Load  V=13800  Ts=Ts
  SSN Interface Block (3ph)3 : ssn_lib/SSN Interface Block (3ph)  nb_phase=3  nb_port=2  p1_type=V-type(Left)  p2_type=V-type (Right)  p3_type=V-type(Left)  p4_type=V-type(Left)  p5_type=V-type(Left)  p6_type=V-type(Left)  p7_type=V-type(Left)  p8_type=V-type(Left)  p9_type=V-type(Left)  p10_type=V-type(Left)  p11_type=V-type(Left)  p12_type=V-type(Left)  p13_type=V-type(Left)  p14_type=V-type(Left)  p15_type=V-type(Left)  p16_type=V-type(Left)  I_port_shunt_resistance=1e9
  "Start_Index " : Constant
  "State " : Constant
  "Stop_Index " : Constant  Value=1800-1
  "Time_Scale_Factor " : Constant
  A_CB_F2 : PMIOPort  Port=1  Side=Right
  B_CB_F2 : PMIOPort  Port=2  Side=Right
  C_CB_F2 : PMIOPort  Port=3  Side=Right
  A_PCC : PMIOPort  Port=4  Side=Left
  B_PCC : PMIOPort  Port=5  Side=Left
  C_PCC : PMIOPort  Port=6  Side=Left
  A_CB_F1 : PMIOPort  Port=7  Side=Left
  B_CB_F1 : PMIOPort  Port=8  Side=Right
  C_CB_F1 : PMIOPort  Port=9  Side=Left
  DATA_OUT : Outport
  wires:
  CB closed/1 -> Bus Creator/1  "Logic_trip"
  Bus Creator/1 -> [cb_c]
  Bus Selector1/1 -> F3_CB_2/1  "<F3_CB_2>"
  LOAD_IN/1 -> OpComm1/1
  OpComm1/1 -> [LOAD_IN]
  [LOAD_IN] -> Bus Selector3/1
  [LOAD_IN] -> Bus Selector5/1
  Bus Selector3/1 -> NONSHEDDABLE/1  "<NONSHEDDABLE>"
  Bus Selector5/1 -> SHEDDABLE/1  "<SHEDDABLE>"
  NONSHEDDABLE/1 -> [LOAD_NONSHEDDABLE]
  SHEDDABLE/1 -> [LOAD_SHEDDABLE]
  [LOAD_SHEDDABLE] -> Bus Creator3/2  "F3_SHEDDABLE"
  [LOAD_NONSHEDDABLE] -> Bus Creator3/1  "F3_NONSHEDDABLE"
  Bus Creator3/1 -> [LOAD_DATA]  "LOAD"
  F3_CB_2/1 -> [F3_CB_2]
  F3_CB_3/1 -> [F3_CB_3]
  [F3_CB_1] -> Bus Creator5/1  "F3_CB_1"
  [F3_CB_3] -> Bus Creator5/3  "F3_CB_3"
  [F3_CB_2] -> Bus Creator5/2  "F3_CB_2"
  Bus Creator5/1 -> [CB_DATA]
  [RELAY_IN] -> Bus Selector1/1
  RELAY_IN/1 -> OpComm1/2
  OpComm1/2 -> [RELAY_IN]
  Bus Selector9/1 -> F3_CB_3/1  "<F3_CB_3>"
  [RELAY_IN] -> Bus Selector9/1
  [cb_c] -> F3_PCC/1
  F3_PCC/1 -> [F3_PCC]
  [F3_PCC] -> Bus Creator5/4  "F3_PCC"
  SC_CMD/1 -> OpComm2/1
  Memory/1 -> DATA_OUT/1
  "Start_Index "/1 -> Mux/3
  "Time_Scale_Factor "/1 -> Mux/5
  "State "/1 -> Mux/1
  Demux2/1 -> OpFromFile/1
  Demux2/4 -> OpFromFile/4
  OpFromFile/2 -> [heat_load]  "Heat Load MBtu/hr"
  Demux2/5 -> OpFromFile/5
  "Repetative "/1 -> Mux/2
  Demux2/3 -> OpFromFile/3
  Demux2/6 -> OpFromFile/6
  Demux2/2 -> OpFromFile/2
  Mux/1 -> Demux2/1
  "Interpolation "/1 -> Mux/6
  "Stop_Index "/1 -> Mux/4
  OpComm2/1 -> Bus Selector15/1
  F3_GCB/1 -> PQFV/1
  PQFV/1 -> Bus Creator6/3  "NG_CHP_GCB"
  HWController_3.5MVA_NGCHP/2(Generator Data) -> Bus Creator6/2  "Gen1_meas"
  HWController_3.5MVA_NGCHP/1(Out1) -> Bus Creator6/1  "CHPData"
  [CHP_SIM_cmds] -> HWController_3.5MVA_NGCHP/2(In2)
  Bus Creator6/1 -> [NG_CHP_DATA]
  [NGCHP_Gen1] -> HWController_3.5MVA_NGCHP/3(HWControllerBias)
  HWController_3.5MVA_NGCHP/3(GCB Control) -> F3_GCB/1
  [heat_load] -> HWController_3.5MVA_NGCHP/1(In1)
  HWCtrl_CMD/1 -> OpComm1/3
  OpComm1/3 -> Bus Selector16/1
  Bus Selector16/1 -> [NGCHP_Gen1]  "<NGCHP_Gen1>"
  Bus Creator2/1 -> Memory/1
  [CB_DATA] -> Bus Creator2/1  "CB_DATA"
  [LOAD_DATA] -> Bus Creator2/2  "LOAD_DATA"
  [NG_CHP_DATA] -> Bus Creator2/3  "NG_CHP_DATA"
  Bus Selector15/1 -> [CHP_SIM_cmds]  "<CHP_SIM_Cmds>"
  Bus Selector2/1 -> F3_CB_1/1  "<F3_CB_1>"
  F3_CB_1/1 -> [F3_CB_1]
  [RELAY_IN] -> Bus Selector2/1
  connections:
  C301/LConn2 -- F3_CB_3/RConn2
  C301/LConn3 -- F3_CB_3/RConn3
  F3_GCB/RConn3 -- C302/RConn3
  F3_GCB/RConn1 -- C302/RConn1
  F3_GCB/RConn2 -- C302/RConn2
  C301/LConn1 -- F3_CB_3/RConn1
  2500 kVA/RConn1 -- A_CB_F2/RConn1
  2500 kVA/RConn3 -- C_CB_F2/RConn1
  2500 kVA/RConn2 -- B_CB_F2/RConn1
  C303/LConn1 -- F3_CB_2/RConn1
  C303/LConn2 -- F3_CB_2/RConn2
  C303/LConn3 -- F3_CB_2/RConn3
  C303/RConn2 -- 2500 kVA/LConn2
  C303/RConn3 -- 2500 kVA/LConn3
  C303/RConn1 -- 2500 kVA/LConn1
  F3_PCC/LConn2 -- B_PCC/RConn1
  F3_PCC/LConn3 -- C_PCC/RConn1
  F3_PCC/LConn1 -- A_PCC/RConn1
  PI-Section2/RConn3 -- F3_GCB/LConn3
  PI-Section2/RConn2 -- F3_GCB/LConn2
  PI-Section2/RConn1 -- F3_GCB/LConn1
  HWController_3.5MVA_NGCHP/RConn2 -- PI-Section2/LConn2
  HWController_3.5MVA_NGCHP/RConn3 -- PI-Section2/LConn3
  HWController_3.5MVA_NGCHP/RConn1 -- PI-Section2/LConn1
  C301/RConn1 -- SHEDDABLE/LConn1
  C301/RConn2 -- SHEDDABLE/LConn2
  C301/RConn3 -- SHEDDABLE/LConn3
  F3_PCC/RConn1 -- C302/LConn1 -- F3_CB_3/LConn1 -- SSN Interface Block (3ph)3/LConn1 -- NONSHEDDABLE/LConn1
  F3_PCC/RConn2 -- F3_CB_3/LConn2 -- SSN Interface Block (3ph)3/LConn2 -- C302/LConn2 -- NONSHEDDABLE/LConn2
  F3_PCC/RConn3 -- C302/LConn3 -- F3_CB_3/LConn3 -- SSN Interface Block (3ph)3/LConn3 -- NONSHEDDABLE/LConn3
  2500 kVA1/RConn1 -- A_CB_F1/RConn1
  2500 kVA1/RConn3 -- C_CB_F1/RConn1
  2500 kVA1/RConn2 -- B_CB_F1/RConn1
  C304/LConn1 -- F3_CB_1/RConn1
  C304/LConn2 -- F3_CB_1/RConn2
  C304/LConn3 -- F3_CB_1/RConn3
  C304/RConn2 -- 2500 kVA1/LConn2
  C304/RConn1 -- 2500 kVA1/LConn1
  C304/RConn3 -- 2500 kVA1/LConn3
  SSN Interface Block (3ph)3/RConn1 -- F3_CB_2/LConn1 -- F3_CB_1/LConn1
  SSN Interface Block (3ph)3/RConn2 -- F3_CB_2/LConn2 -- F3_CB_1/LConn2
  SSN Interface Block (3ph)3/RConn3 -- F3_CB_2/LConn3 -- F3_CB_1/LConn3

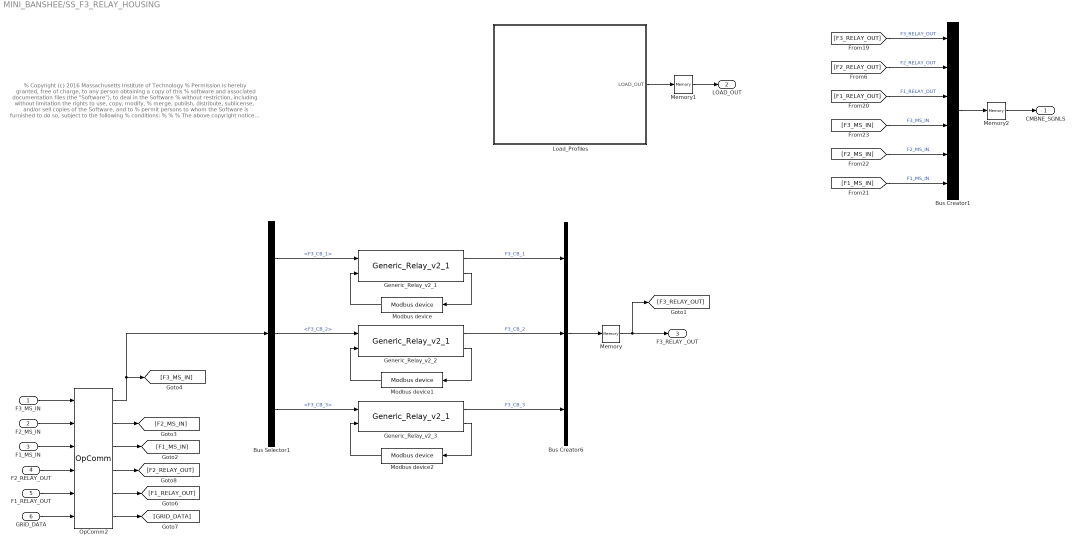
== system MINI_BANSHEE/SS_F3_RELAY_HOUSING ==
  note: % Copyright (c) 2016 Massachusetts Institute of Technology
      | % Permission is hereby granted, free of charge, to any person obtaining a copy of this
      | % software and associated documentation files (the "Software"), to deal in the Software
      | % without restriction, including without limitation the rights to use, copy, modify,
      | % merge, publish, distribute, sublicense, and/or sell copies of the Software, and to
      | % permit persons to whom the Software is furnished to do so, subject to the following
      | % conditions:
      | %
      | %
      | % The above copyright notice and this permission notice shall be included in
      | % all copies or substantial portions of the Software.
      | %
      | % THE SOFTWARE IS PROVIDED "AS IS", WITHOUT WARRANTY OF ANY KIND, EXPRESS OR IMPLIED,
      | % INCLUDING BUT NOT LIMITED TO THE WARRANTIES OF MERCHANTABILITY, FITNESS FOR A
      | % PARTICULAR PURPOSE AND NONINFRINGEMENT. IN NO EVENT SHALL THE AUTHORS OR COPYRIGHT
      | % HOLDERS BE LIABLE FOR ANY CLAIM, DAMAGES OR OTHER LIABILITY, WHETHER IN AN ACTION
      | % OF CONTRACT, TORT OR OTHERWISE, ARISING FROM, OUT OF OR IN CONNECTION WITH THE
      | % SOFTWARE OR THE USE OR OTHER DEALINGS IN THE SOFTWARE.
      | %
      | %
      | %%
  F3_MS_IN : Inport
  F2_MS_IN : Inport  Port=2
  F1_MS_IN : Inport  Port=3
  F2_RELAY_OUT : Inport  Port=4
  F1_RELAY_OUT : Inport  Port=5
  GRID_DATA : Inport  Port=6
  Bus Creator1 : BusCreator  Inputs=6
  Bus Creator6 : BusCreator  Inputs=3
  Bus Selector1 : BusSelector  OutputSignals=CB_DATA.F3_CB_1,CB_DATA.F3_CB_2,CB_DATA.F3_CB_3
  Generic_Relay_v2_1 : relay_modbus_lib/Generic_Relay_v2_1  Ts=Ts  relay_settings=[F3(1,:)]
  Generic_Relay_v2_2 : relay_modbus_lib/Generic_Relay_v2_1  Ts=Ts  relay_settings=[F3(2,:)]
  Generic_Relay_v2_3 : relay_modbus_lib/Generic_Relay_v2_1  Ts=Ts  relay_settings=[F3(3,:)]
  Load_Profiles : Subsystem
  Memory : Memory
  Memory1 : Memory
  Memory2 : Memory
  Modbus device : rtio_generic_modbus/Modbus device  conf_name=F3_relay_cfg1.opal  conf_name_mask=F3_relay_cfg1.xls  sample_time=Ts
  Modbus device1 : rtio_generic_modbus/Modbus device  conf_name=F3_relay_cfg2.opal  conf_name_mask=F3_relay_cfg2.xls  sample_time=Ts
  Modbus device2 : rtio_generic_modbus/Modbus device  conf_name=F3_relay_cfg3.opal  conf_name_mask=F3_relay_cfg3.xls  sample_time=Ts
  OpComm2 : rtlab/OpComm  nbport=6  groupe_acq=1  subsys_rate=0  st=0  Synchronization=on  Interpolation=on  Threshold=1.0  Missed_Data=off  Sim_Time=off  Samples=off  dynSigOut=off  from_console=0  warning_done=off  writeOpCommFile=off  Offset=off
  CMBNE_SGNLS : Outport
  LOAD_OUT : Outport  Port=2
  F3_RELAY _OUT : Outport  Port=3
  wires:
  Load_Profiles/1(LOAD_OUT) -> Memory1/1
  OpComm2/1 -> Bus Selector1/1, [F3_MS_IN]
  Generic_Relay_v2_1/2 -> Modbus device/1
  Modbus device/1 -> Generic_Relay_v2_1/2
  Generic_Relay_v2_2/2 -> Modbus device1/1
  Modbus device1/1 -> Generic_Relay_v2_2/2
  Modbus device2/1 -> Generic_Relay_v2_3/2
  Generic_Relay_v2_3/2 -> Modbus device2/1
  F3_MS_IN/1 -> OpComm2/1
  Bus Selector1/1 -> Generic_Relay_v2_1/1  "<F3_CB_1>"
  Bus Selector1/2 -> Generic_Relay_v2_2/1  "<F3_CB_2>"
  Bus Selector1/3 -> Generic_Relay_v2_3/1  "<F3_CB_3>"
  Generic_Relay_v2_1/1 -> Bus Creator6/1  "F3_CB_1"
  Generic_Relay_v2_2/1 -> Bus Creator6/2  "F3_CB_2"
  Generic_Relay_v2_3/1 -> Bus Creator6/3  "F3_CB_3"
  Bus Creator6/1 -> Memory/1
  Memory/1 -> [F3_RELAY_OUT], F3_RELAY _OUT/1
  Memory1/1 -> LOAD_OUT/1
  F2_RELAY_OUT/1 -> OpComm2/4
  F1_RELAY_OUT/1 -> OpComm2/5
  OpComm2/4 -> [F2_RELAY_OUT]
  OpComm2/5 -> [F1_RELAY_OUT]
  OpComm2/2 -> [F2_MS_IN]
  OpComm2/3 -> [F1_MS_IN]
  F2_MS_IN/1 -> OpComm2/2
  F1_MS_IN/1 -> OpComm2/3
  OpComm2/6 -> [GRID_DATA]
  GRID_DATA/1 -> OpComm2/6
  Memory2/1 -> CMBNE_SGNLS/1
  Bus Creator1/1 -> Memory2/1
  [F1_MS_IN] -> Bus Creator1/6  "F1_MS_IN"
  [F2_RELAY_OUT] -> Bus Creator1/2  "F2_RELAY_OUT"
  [F1_RELAY_OUT] -> Bus Creator1/3  "F1_RELAY_OUT"
  [F3_RELAY_OUT] -> Bus Creator1/1  "F3_RELAY_OUT"
  [F3_MS_IN] -> Bus Creator1/4  "F3_MS_IN"
  [F2_MS_IN] -> Bus Creator1/5  "F2_MS_IN"
